simulink model "Thirtybussys_pv"  (R2023b)
settings: Solver=VariableStepAuto  StartTime=0.0  StopTime=1  RelTol=1e-3
undefined symbols (not defined in the file): A, B, C, Dd, j, to, V2G
libraries: spsFourierLib x60, spsThreePhaseSeriesRLCBranchLib x41, spsThreePhaseVIMeasurementLib x31, spsPower3phInstantaneousLib x30, spsThreePhaseSeriesRLCLoadLib x21, spsThreePhaseSourceLib x6, spsThreePhaseTransformerTwoWindingsLib x6, spsControlledCurrentSourceLib x2, spsSeriesRLCBranchLib x2, spsVoltageMeasurementLib x2, simulink x2, spsPower3phPhasorLib x1
(part 3 of 3)

== system Thirtybussys_pv/Subsystem30/Subsystem23 ==
  In1 : Inport
  Add : Sum  Inputs=+++
  Demux : Demux  Outputs=3
  Fourier : spsFourierLib/Fourier  Freq=60  n=1  InInit=[0, 0]  Ts=0
  Gain : Gain
  Scope : Scope
  Outport : Outport  VectorParamsAs1DForOutWhenUnconnected=off
  wires:
  Demux/3 -> Add/3
  Add/1 -> Gain/1
  Gain/1 -> Outport/1
  Fourier/2 -> Scope/1
  In1/1 -> Fourier/1
  Demux/2 -> Add/2
  Fourier/1 -> Demux/1
  Demux/1 -> Add/1

== system Thirtybussys_pv/Subsystem30/Subsystem24 ==
  In1 : Inport
  Add : Sum  Inputs=+++
  Demux : Demux  Outputs=3
  Fourier : spsFourierLib/Fourier  Freq=60  n=1  InInit=[0, 0]  Ts=0
  Gain : Gain
  Scope : Scope
  Outport : Outport  VectorParamsAs1DForOutWhenUnconnected=off
  wires:
  Demux/1 -> Add/1
  Fourier/1 -> Demux/1
  Demux/2 -> Add/2
  In1/1 -> Fourier/1
  Fourier/2 -> Scope/1
  Gain/1 -> Outport/1
  Add/1 -> Gain/1
  Demux/3 -> Add/3

== system Thirtybussys_pv/Subsystem30/Subsystem25 ==
  In1 : Inport
  Add : Sum  Inputs=+++
  Demux : Demux  Outputs=3
  Fourier : spsFourierLib/Fourier  Freq=60  n=1  InInit=[0, 0]  Ts=0
  Gain : Gain
  Scope : Scope
  Outport : Outport  VectorParamsAs1DForOutWhenUnconnected=off
  wires:
  Demux/3 -> Add/3
  Add/1 -> Gain/1
  Gain/1 -> Outport/1
  Fourier/2 -> Scope/1
  In1/1 -> Fourier/1
  Demux/2 -> Add/2
  Fourier/1 -> Demux/1
  Demux/1 -> Add/1

== system Thirtybussys_pv/Subsystem30/Subsystem26 ==
  In1 : Inport
  Add : Sum  Inputs=+++
  Demux : Demux  Outputs=3
  Fourier : spsFourierLib/Fourier  Freq=60  n=1  InInit=[0, 0]  Ts=0
  Gain : Gain
  Scope : Scope
  Outport : Outport  VectorParamsAs1DForOutWhenUnconnected=off
  wires:
  Demux/3 -> Add/3
  Add/1 -> Gain/1
  Gain/1 -> Outport/1
  Fourier/2 -> Scope/1
  In1/1 -> Fourier/1
  Demux/2 -> Add/2
  Fourier/1 -> Demux/1
  Demux/1 -> Add/1

== system Thirtybussys_pv/Subsystem30/Subsystem27 ==
  In1 : Inport
  Add : Sum  Inputs=+++
  Demux : Demux  Outputs=3
  Fourier : spsFourierLib/Fourier  Freq=60  n=1  InInit=[0, 0]  Ts=0
  Gain : Gain
  Scope : Scope
  Outport : Outport  VectorParamsAs1DForOutWhenUnconnected=off
  wires:
  Demux/1 -> Add/1
  Fourier/1 -> Demux/1
  Demux/2 -> Add/2
  In1/1 -> Fourier/1
  Fourier/2 -> Scope/1
  Gain/1 -> Outport/1
  Add/1 -> Gain/1
  Demux/3 -> Add/3

== system Thirtybussys_pv/Subsystem30/Subsystem28 ==
  In1 : Inport
  Add : Sum  Inputs=+++
  Demux : Demux  Outputs=3
  Fourier : spsFourierLib/Fourier  Freq=60  n=1  InInit=[0, 0]  Ts=0
  Gain : Gain
  Scope : Scope
  Outport : Outport  VectorParamsAs1DForOutWhenUnconnected=off
  wires:
  Demux/1 -> Add/1
  Fourier/1 -> Demux/1
  Demux/2 -> Add/2
  In1/1 -> Fourier/1
  Fourier/2 -> Scope/1
  Gain/1 -> Outport/1
  Add/1 -> Gain/1
  Demux/3 -> Add/3

== system Thirtybussys_pv/Subsystem30/Subsystem29 ==
  In1 : Inport
  Add : Sum  Inputs=+++
  Demux : Demux  Outputs=3
  Fourier : spsFourierLib/Fourier  Freq=60  n=1  InInit=[0, 0]  Ts=0
  Gain : Gain
  Scope : Scope
  Outport : Outport  VectorParamsAs1DForOutWhenUnconnected=off
  wires:
  Demux/3 -> Add/3
  Add/1 -> Gain/1
  Gain/1 -> Outport/1
  Fourier/2 -> Scope/1
  In1/1 -> Fourier/1
  Demux/2 -> Add/2
  Fourier/1 -> Demux/1
  Demux/1 -> Add/1

== system Thirtybussys_pv/Subsystem30/Subsystem3 ==
  In1 : Inport
  Add : Sum  Inputs=+++
  Demux : Demux  Outputs=3
  Fourier : spsFourierLib/Fourier  Freq=60  n=1  InInit=[0, 0]  Ts=0
  Gain : Gain
  Scope : Scope
  Outport : Outport  VectorParamsAs1DForOutWhenUnconnected=off
  wires:
  Demux/3 -> Add/3
  Add/1 -> Gain/1
  Gain/1 -> Outport/1
  Fourier/2 -> Scope/1
  In1/1 -> Fourier/1
  Demux/2 -> Add/2
  Fourier/1 -> Demux/1
  Demux/1 -> Add/1

== system Thirtybussys_pv/Subsystem30/Subsystem4 ==
  In1 : Inport
  Add : Sum  Inputs=+++
  Demux : Demux  Outputs=3
  Fourier : spsFourierLib/Fourier  Freq=60  n=1  InInit=[0, 0]  Ts=0
  Gain : Gain
  Scope : Scope
  Outport : Outport  VectorParamsAs1DForOutWhenUnconnected=off
  wires:
  Demux/1 -> Add/1
  Fourier/1 -> Demux/1
  Demux/2 -> Add/2
  In1/1 -> Fourier/1
  Fourier/2 -> Scope/1
  Gain/1 -> Outport/1
  Add/1 -> Gain/1
  Demux/3 -> Add/3

== system Thirtybussys_pv/Subsystem30/Subsystem5 ==
  In1 : Inport
  Add : Sum  Inputs=+++
  Demux : Demux  Outputs=3
  Fourier : spsFourierLib/Fourier  Freq=60  n=1  InInit=[0, 0]  Ts=0
  Gain : Gain
  Scope : Scope
  Outport : Outport  VectorParamsAs1DForOutWhenUnconnected=off
  wires:
  Demux/3 -> Add/3
  Add/1 -> Gain/1
  Gain/1 -> Outport/1
  Fourier/2 -> Scope/1
  In1/1 -> Fourier/1
  Demux/2 -> Add/2
  Fourier/1 -> Demux/1
  Demux/1 -> Add/1

== system Thirtybussys_pv/Subsystem30/Subsystem6 ==
  In1 : Inport
  Add : Sum  Inputs=+++
  Demux : Demux  Outputs=3
  Fourier : spsFourierLib/Fourier  Freq=60  n=1  InInit=[0, 0]  Ts=0
  Gain : Gain
  Scope : Scope
  Outport : Outport  VectorParamsAs1DForOutWhenUnconnected=off
  wires:
  Demux/3 -> Add/3
  Add/1 -> Gain/1
  Gain/1 -> Outport/1
  Fourier/2 -> Scope/1
  In1/1 -> Fourier/1
  Demux/2 -> Add/2
  Fourier/1 -> Demux/1
  Demux/1 -> Add/1

== system Thirtybussys_pv/Subsystem30/Subsystem7 ==
  In1 : Inport
  Add : Sum  Inputs=+++
  Demux : Demux  Outputs=3
  Fourier : spsFourierLib/Fourier  Freq=60  n=1  InInit=[0, 0]  Ts=0
  Gain : Gain
  Scope : Scope
  Outport : Outport  VectorParamsAs1DForOutWhenUnconnected=off
  wires:
  Demux/1 -> Add/1
  Fourier/1 -> Demux/1
  Demux/2 -> Add/2
  In1/1 -> Fourier/1
  Fourier/2 -> Scope/1
  Gain/1 -> Outport/1
  Add/1 -> Gain/1
  Demux/3 -> Add/3

== system Thirtybussys_pv/Subsystem30/Subsystem8 ==
  In1 : Inport
  Add : Sum  Inputs=+++
  Demux : Demux  Outputs=3
  Fourier : spsFourierLib/Fourier  Freq=60  n=1  InInit=[0, 0]  Ts=0
  Gain : Gain
  Scope : Scope
  Outport : Outport  VectorParamsAs1DForOutWhenUnconnected=off
  wires:
  Demux/1 -> Add/1
  Fourier/1 -> Demux/1
  Demux/2 -> Add/2
  In1/1 -> Fourier/1
  Fourier/2 -> Scope/1
  Gain/1 -> Outport/1
  Add/1 -> Gain/1
  Demux/3 -> Add/3

== system Thirtybussys_pv/Subsystem30/Subsystem9 ==
  In1 : Inport
  Add : Sum  Inputs=+++
  Demux : Demux  Outputs=3
  Fourier : spsFourierLib/Fourier  Freq=60  n=1  InInit=[0, 0]  Ts=0
  Gain : Gain
  Scope : Scope
  Outport : Outport  VectorParamsAs1DForOutWhenUnconnected=off
  wires:
  Demux/3 -> Add/3
  Add/1 -> Gain/1
  Gain/1 -> Outport/1
  Fourier/2 -> Scope/1
  In1/1 -> Fourier/1
  Demux/2 -> Add/2
  Fourier/1 -> Demux/1
  Demux/1 -> Add/1

== system Thirtybussys_pv/PV Farm 8 MW/PV Farm/Avoid division by zero ==
  I : Inport
  Complex to Magnitude-Angle : ComplexToMagnitudeAngle
  Magnitude-Angle to Complex : MagnitudeAngleToComplex
  Saturation1 : Saturate  UpperLimit=inf  LowerLimit=1e-6
  O : Outport  VectorParamsAs1DForOutWhenUnconnected=off
  wires:
  Complex to Magnitude-Angle/2 -> Magnitude-Angle to Complex/2
  Magnitude-Angle to Complex/1 -> O/1
  Complex to Magnitude-Angle/1 -> Saturation1/1
  Saturation1/1 -> Magnitude-Angle to Complex/1
  I/1 -> Complex to Magnitude-Angle/1

== system Thirtybussys_pv/PV Farm 8 MW/PV Farm/Break Alg. Loop 1 ==
  In : Inport
  Complex to Real-Imag : ComplexToRealImag
  Real-Imag to Complex : RealImagToComplex
  imag : Subsystem  mask(Transfer Function with Initial Outputs){N=[1], D=[to  1], Y0=0, U0=0}
      mask prompts: N "Numerator:"; D "Denominator:"; Y0 "Initial output:"; U0 "Initial input:"
      mask help: Vector expressions for numerator, and denominator. Coefficients are in descending powers of s.
      mask init:
      | [A,B,C,Dd]=tf2ss(N,D);if (isempty(Y0));[m,n]=size(A);X0=zeros(1,m); end; if (isempty(U0));[m,p]=size(B);U0=zeros(1,p);end;X0=getxo(A,B,C,Dd,U0,Y0,0);
      mask Help: Specify the initial output for the transfer function.  An optimization routine attempts to determine the appropriate initial states so that the specified initial output is achieved.  For more details, see the m-file getxo.m
      mask Display: dpoly(N,D,'s')
  real : Subsystem  mask(Transfer Function with Initial Outputs){N=[1], D=[to 1], Y0=0, U0=0}
      mask prompts: N "Numerator:"; D "Denominator:"; Y0 "Initial output:"; U0 "Initial input:"
      mask help: Vector expressions for numerator, and denominator. Coefficients are in descending powers of s.
      mask init:
      | [A,B,C,Dd]=tf2ss(N,D);if (isempty(Y0));[m,n]=size(A);X0=zeros(1,m); end; if (isempty(U0));[m,p]=size(B);U0=zeros(1,p);end;X0=getxo(A,B,C,Dd,U0,Y0,0);
      mask Help: Specify the initial output for the transfer function.  An optimization routine attempts to determine the appropriate initial states so that the specified initial output is achieved.  For more details, see the m-file getxo.m
      mask Display: dpoly(N,D,'s')
  Out : Outport  VectorParamsAs1DForOutWhenUnconnected=off
  wires:
  Complex to Real-Imag/1 -> real/1(In1)
  Complex to Real-Imag/2 -> imag/1(In1)
  In/1 -> Complex to Real-Imag/1
  Real-Imag to Complex/1 -> Out/1
  real/1(Out1) -> Real-Imag to Complex/1
  imag/1(Out1) -> Real-Imag to Complex/2

== system Thirtybussys_pv/PV Farm 8 MW/PV Farm/Break Alg. Loop 1/imag ==
  In1 : Inport
  State Space : StateSpace  A=A  B=B  C=C  D=Dd  InitialCondition=X0
  Out1 : Outport  InitialOutput=0  VectorParamsAs1DForOutWhenUnconnected=off
  wires:
  State Space/1 -> Out1/1
  In1/1 -> State Space/1

== system Thirtybussys_pv/PV Farm 8 MW/PV Farm/Break Alg. Loop 1/real ==
  In1 : Inport
  State Space : StateSpace  A=A  B=B  C=C  D=Dd  InitialCondition=X0
  Out1 : Outport  InitialOutput=0  VectorParamsAs1DForOutWhenUnconnected=off
  wires:
  State Space/1 -> Out1/1
  In1/1 -> State Space/1
